simulink model "CalculatorSF_Task"  (R2021a)
settings: Solver=FixedStepDiscrete  StartTime=0.0  StopTime=10.0  RelTol=1e-3
settings Model: Creator=Mohamed Elomda  LastModifiedBy=Mohamed Elomda
settings OptimizationCC: DefaultParameterBehavior=Inlined  EnhancedBackFolding=on  PassReuseOutputArgsAs=Individual arguments  ZeroExternalMemoryAtStartup=off  ZeroInternalMemoryAtStartup=off  OptimizeBlockOrder=speed  DifferentSizesBufferReuse=on  OptimizationCustomize=off  EfficientTunableParamExpr=on
settings DebuggingCC: UnderspecifiedInitializationDetection=Classic  MergeDetectMultiDrivingBlocksExec=none  ParameterTunabilityLossMsg=error
settings ModelReferenceCC: PropagateSignalLabelsOutOfModel=off
settings SFSimCC: MATLABDynamicMemAlloc=off
settings RTWCC: SystemTargetFile=ert.tlc  GenCodeOnly=on  TemplateMakefile=ert_default_tmf  GenerateReport=on  LaunchReport=on
settings CodeAppCC: ForceParamTrailComments=on  IgnoreCustomStorageClasses=off  OperatorAnnotations=on  SimulinkDataObjDesc=on  SFDataObjDesc=on  InsertBlockDesc=on
settings ERTTargetCC: TargetLangStandard=C99 (ISO)  GenerateSampleERTMain=on  InlinedParameterPlacement=NonHierarchical  ERTCustomFileTemplate=example_file_process.tlc

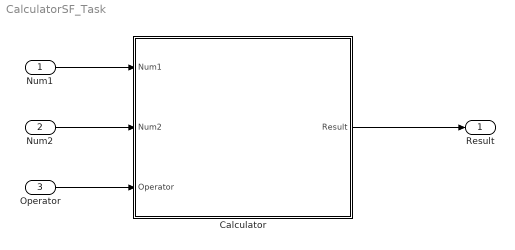
== system CalculatorSF_Task ==
  Num1 : Inport
  Num2 : Inport  Port=2
  Operator : Inport  Port=3
  Calculator : Stateflow chart  TreatAsAtomicUnit=on
      settings: RTWSystemCode=Reusable function  RTWFcnNameOpts=Use subsystem name  RTWFileNameOpts=Use subsystem name  PortSchema="{\"entries\":[{\"content\":{\"sides\":[{\"content\":{\"connectorIds\":[\"In2\",\"In1\",\"In3\"]},\"type\":\"ConnectorPlacement.EquallySpacedRectSide\",\"uuid\":\"906ca186-096a-4428-b569-5a280e1bb027\"},{\"content\":{\"connectorIds\":[\"Out1\"],\"side\":\"RIGHT\"},\"type\":\"ConnectorPlacement.EquallySpacedRectSide\",\"uuid\":\"7a5f9e6f-72c9-4f68-abd8-927e021c8263\"},{\"content\":{\"connectorIds\":[],\"side\":\"TOP\"},\"type\":\"ConnectorPlacement.EquallySpacedRectSide\",\"uuid\":\"8c9e7eb6-71a6-4cdd-b4f0-9b3eb2fc8446\"}]},\"type\":\"ConnectorPlacement.EquallySpacedConnector\",\"uuid\":\"c357dc16-4e9f-4627-b165-711c27a7154f\"}],\"packageUris\":[\"http://schema.mathworks.com/mf0/Connector/R2020b\"],\"version\":\"1.0\"}"
  Result : Outport
  wires:
  Calculator/1(Result) -> Result/1
  Operator/1 -> Calculator/3(Operator)
  Num2/1 -> Calculator/1(Num2)
  Num1/1 -> Calculator/2(Num1)

== stateflow chart CalculatorSF_Task/Calculator ==
  state add(N1,N2) [function]
    (default) -> (junction 24) : {Result = N1 + N2;}
  state Calculator
    (default) -> (junction 49) : % Calculation
    (junction 49) -> (junction 50) [order 1] : [Operator == 0]
    (junction 49) -> (junction 51) [order 2]
    (junction 50) -> (junction 58) : {add(Num1,Num2);}
    (junction 51) -> (junction 52) [order 1] : [Operator == 1]
    (junction 51) -> (junction 53) [order 2]
    (junction 52) -> (junction 57) : {sub(Num1,Num2);}
    (junction 53) -> (junction 54) [order 1] : [Operator == 2]
    (junction 53) -> (junction 55) [order 2] : {divide(Num1,Num2);}
    (junction 54) -> (junction 56) : {multiply(Num1,Num2);}
    (junction 56) -> (junction 55)
    (junction 57) -> (junction 56)
    (junction 58) -> (junction 57)
    (junction 55) -> (junction 59)
  state sub(N1,N2) [function]
    (default) -> (junction 5) : {Result = N1 - N2;}
  state multiply(N1,N2) [function]
    (default) -> (junction 8) : {Result = N1 * N2;}
  state divide(N1,N2) [function]
    (default) -> (junction 14)
    (junction 14) -> (junction 61) [order 1] : [N2 == 0]
    (junction 61) -> (junction 65) : {Result = -1;}
    (junction 14) -> (junction 65) [order 2] : {Result = N1 / N2;}
  (default) -> Calculator
  data: N1 function_input; N2 function_input; N1 function_input; N2 function_input; N1 function_input; N2 function_input; N1 function_input; N2 function_input; Num2 input; Num1 input; Operator input double; Result output
